simulink model "drive_to_point"  (Simulink 8.9)
settings: Solver=ode45  StartTime=0.0  StopTime=15.0  RelTol=1e-3  EnableMultiTasking=on
values from neighbouring files (symbols this model uses):
  xg = [x,y]    [ComplexEngineeringProblem.m]
libraries: roblocks x2
settings Model: Creator=pic  LastModifiedBy=Abdullah
settings DataIOCC: LimitDataPoints=off  ReturnWorkspaceOutputs=on
settings OptimizationCC: ExpressionDepthLimit=2147483647
settings DebuggingCC: StrictBusMsg=Warning

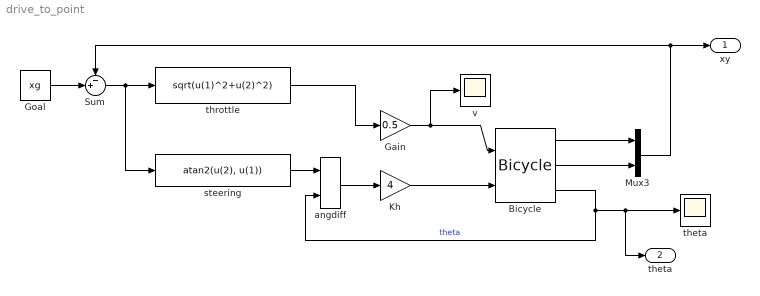
== system drive_to_point ==
  Bicycle : roblocks/Dynamics/Bicycle  accel=1  vlim=1  alim=1  L=1  x0=x0  handbrake=0
  Gain : Gain  Gain=0.5
  Goal : Constant  Value=xg
  Kh : Gain  Gain=4
  Mux3 : Mux  Inputs=2
  Sum : Sum  Inputs=-+|
  angdiff : roblocks/Trajectory/angdiff
  steering : Fcn  Expr=atan2(u(2), u(1))
  theta : Scope
  throttle : Fcn  Expr=sqrt(u(1)^2+u(2)^2)
  v : Scope
  xy : Outport
  "theta " : Outport  Port=2
  wires:
  Bicycle/1 -> Mux3/1
  Bicycle/2 -> Mux3/2
  Mux3/1 -> xy/1, Sum/1
  Sum/1 -> throttle/1, steering/1
  throttle/1 -> Gain/1
  steering/1 -> angdiff/1
  Bicycle/3 -> theta/1, "theta "/1, angdiff/2  "theta"
  angdiff/1 -> Kh/1
  Gain/1 -> v/1, Bicycle/1
  Goal/1 -> Sum/2
  Kh/1 -> Bicycle/2
